simulink model "Compensansion"  (R2023b)
settings: Solver=VariableStepAuto  StartTime=0.0  StopTime=10.0  RelTol=1e-3
InitFcn:
  | %% Geófono SM-24
  | m   = 0.011;
  | fn  = 10;
  | wn  = 2*pi*fn;
  | k   = m*wn^2;
  | h0  = 0.25;
  | G   = 28.8;
  | d   = 2*m*h0*wn;
  | R_s = 375;
  | 
  | Hg_an = [0, -G, 0];
  | Hg_ad = [1, 2*h0*wn, wn^2];
  | 
  | %% Parámetros del compensador
  | fLow    = 1;
  | wLow    = 2*pi*fLow;
  | h1      = wn/(2*wLow);   % zeta del compensador = 25
  | 
  | Ra_sk = 40e3;
  | Rb_sk = 600e3;
  | Rf_sk = 50e3;
  | C1_sk = 2.2e-6;
  | C2_sk = 3.3e-6;
  | R1_sk = 120e3;
  | R2_sk = 1e3;
  | K_u   = 120e3/100e3;
  | 
  | %% FT del Sallen-Key (lo que implementa el circuito real)
  | K_sk  = 1 + Rb_sk/Ra_sk;   % ganancia interna = 16
  | 
  | Hbpn = [0, K_sk/(R1_sk*C1_sk), 0];  % numerador SK real
  | 
  | Hbpd = [1, ...
  |     1/(R1_sk*C1_sk) + 1/(R2_sk*C1_sk) + 1/(R2_sk*C2_sk) - Rb_sk/(Ra_sk*Rf_sk*C1_sk), ...
  |     (R1_sk + Rf_sk)/(R1_sk*Rf_sk*R2_sk*C1_sk*C2_sk)];
  | 
  | %% Verificación: ¿el SK aproxima bien los coeficientes de H_comp?
  | % H_comp denominador ideal: [1, 2*h1*wn, wn^2]
  | w0_sk   = sqrt(Hbpd(3));
  | bw_sk   = Hbpd(2);
  | zeta_sk = bw_sk/(2*w0_sk);
  | 
  | fprintf('=== Verificación SK ===\n');
  | fprintf('w0  SK    = %.4f rad/s  |  target = %.4f\n', w0_sk, wn);
  | fprintf('zeta SK   = %.4f        |  target = %.4f (h1)\n', zeta_sk, h1);
  | fprintf('f0  SK    = %.4f Hz     |  target = %.4f\n', w0_sk/(2*pi), fn);
  | 
  | %% Ganancia K_bp necesaria para escalar el numerador del SK
  | % al numerador ideal de H_comp: 2*(h1-h0)*wn*s
  | coef_s_ideal = 2*(h1 - h0)*wn;      % coeficiente de s en H_comp
  | coef_s_sk    = K_sk/(R1_sk*C1_sk);  % coeficiente de s que entrega el SK
  | 
  | K_bp = 91e3/4.7e3;
  | 
  | fprintf('\n=== Ganancias ===\n');
  | fprintf('K_sk       = %.2f\n', K_sk);
  | fprintf('coef_s_ideal = %.4f\n', coef_s_ideal);
  | fprintf('coef_s_sk    = %.4f\n', coef_s_sk);
  | fprintf('K_bp         = %.6f  (ganancia etapa post-SK)\n', K_bp);
  | 
  | %% FT total del bloque BP escalado
  | % = K_bp * Hbp(s)
  | Hbp_num_escalado = K_bp * Hbpn;
  | 
  | %% Desacople
  | R_d = 10e6;
  | C_d = 10e-6;
  | Hd_n = [1,0];
  | Hd_d = [1,1/(R_d*C_d)];
  | 
  | %% Filtrado Analogico
  | R_TIA = 1000e3;
  | C_TIA = 4.6e-12;
  | C_f   = 820e-12;
  | R_gain = 10e3;
  | R_filter = 470e3;
  | C_filter = 2e-9;
  | 
  | s = tf([1,0],[0,1]);
  | Hfa = ( 1+(R_TIA/R_gain)/(1+R_TIA*(C_TIA+C_f)*s))/(1+R_filter*C_filter*s);
  | Hfa_d = Hfa.Denominator;
  | Hfa_n = Hfa.Numerator;
settings Model: Creator=elias  LastModifiedBy=elias

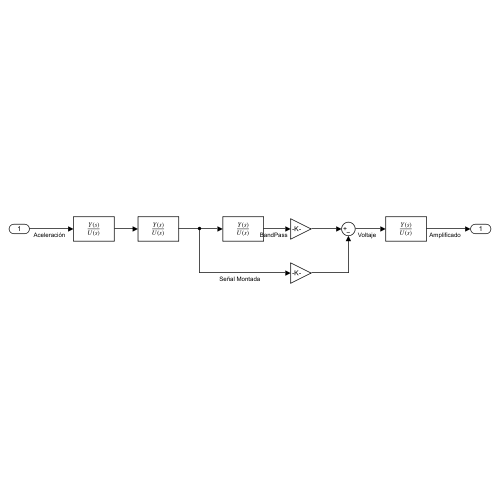
[thumbnail: Simulink's stored preview of the top-level diagram]
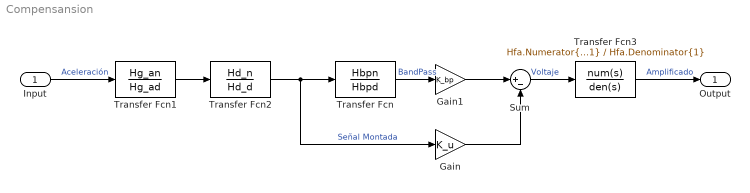
== system Compensansion ==
  Input : Inport
  Gain : Gain  Gain=K_u
  Gain1 : Gain  Gain=K_bp
  Sum : Sum  Inputs=|+-
  Transfer Fcn : TransferFcn  Numerator=Hbpn  Denominator=Hbpd
  Transfer Fcn1 : TransferFcn  Numerator=Hg_an  Denominator=Hg_ad
  Transfer Fcn2 : TransferFcn  Numerator=Hd_n  Denominator=Hd_d
  Transfer Fcn3 : TransferFcn  Numerator=Hfa.Numerator{1}  Denominator=Hfa.Denominator{1}
  Output : Outport
  wires:
  Transfer Fcn/1 -> Gain1/1  "BandPass"
  Sum/1 -> Transfer Fcn3/1  "Voltaje"
  Input/1 -> Transfer Fcn1/1  "Aceleración"
  Gain/1 -> Sum/2
  Gain1/1 -> Sum/1
  Transfer Fcn1/1 -> Transfer Fcn2/1
  Transfer Fcn2/1 -> Transfer Fcn/1, Gain/1  "Señal Montada"
  Transfer Fcn3/1 -> Output/1  "Amplificado"
